simulink model "Example2"  (R2024b)
settings: Solver=FixedStepAuto  StartTime=0.0  StopTime=300  FixedStep=0.01  RelTol=1e-3
settings Model: Creator=aqx  LastModifiedBy=aqx
settings ModelReferenceCC: EnableRefExpFcnMdlSchedulingChecks=on
settings RTWCC: GPUComputeCapability=3.5

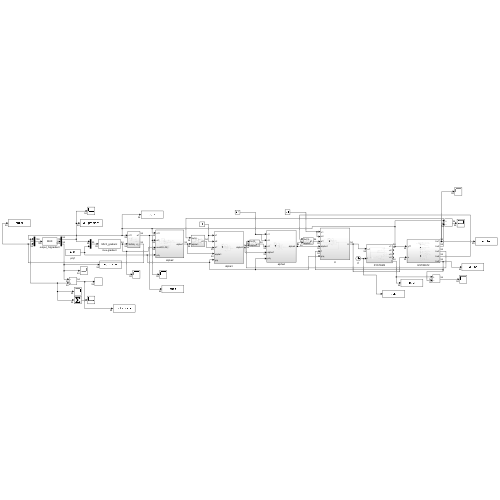
[thumbnail: Simulink's stored preview of the top-level diagram]
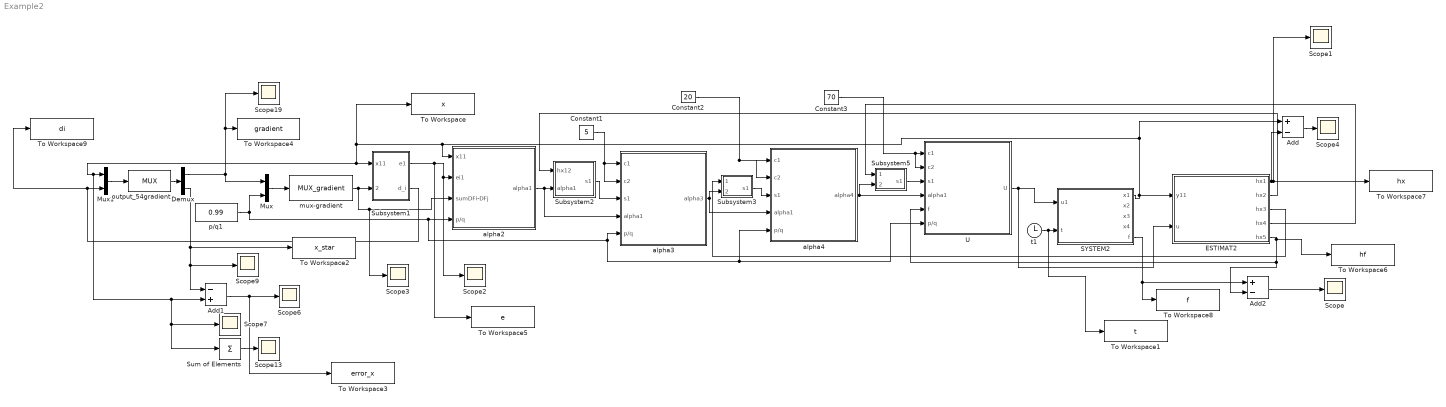
== system Example2 ==
  Add : Sum  Inputs=+-
  Add1 : Sum  Inputs=-+
  Add2 : Sum  Inputs=+-
  Constant1 : Constant  Value=5
  Constant2 : Constant  Value=20
  Constant3 : Constant  Value=70
  Demux : Demux  Outputs=2
  ESTIMAT2 : Subsystem
  Mux : Mux  Inputs=2
  Mux1 : Mux  Inputs=2
  SYSTEM2 : Subsystem
  Scope{,1..4,6..7,9,13,19} (10 alike) : Scope
  Subsystem1 : Subsystem
  Subsystem2 : Subsystem
  Subsystem3 : Subsystem
  Subsystem5 : Subsystem
  Sum of Elements : Sum  Inputs=+
  To Workspace : ToWorkspace  VariableName=x  SampleTime=-1
  To Workspace1 : ToWorkspace  VariableName=t  SampleTime=-1
  To Workspace2 : ToWorkspace  VariableName=x_star  SampleTime=-1
  To Workspace3 : ToWorkspace  VariableName=error_x  SampleTime=-1
  To Workspace4 : ToWorkspace  VariableName=gradient  SampleTime=-1
  To Workspace5 : ToWorkspace  VariableName=e  SampleTime=-1
  To Workspace6 : ToWorkspace  VariableName=hf  SampleTime=-1
  To Workspace7 : ToWorkspace  VariableName=hx  SampleTime=-1
  To Workspace8 : ToWorkspace  VariableName=f  SampleTime=-1
  To Workspace9 : ToWorkspace  VariableName=di  SampleTime=-1
  U : Subsystem
  alpha2 : Subsystem
  alpha3 : Subsystem
  alpha4 : Subsystem
  mux-gradient : S-Function  FunctionName=MUX_gradient  SFunctionDeploymentMode=off  EnableBusSupport=off
  output_54gradient : S-Function  FunctionName=MUX  SFunctionDeploymentMode=off  EnableBusSupport=off
  p/q1 : Constant  Value=0.99
  t1 : Clock
  wires:
  Mux/1 -> mux-gradient/1
  p/q1/1 -> U/6(p/q), alpha4/5(p/q), alpha3/5(p/q), alpha2/4(p/q), Mux/2
  mux-gradient/1 -> Scope3/1, alpha2/3(sumDFi-DFj), Subsystem1/2(SUMi-j)
  Subsystem1/1(e1) -> Scope2/1, alpha2/2(ei1), To Workspace5/1
  alpha2/1(alpha1) -> alpha3/4(alpha1), Subsystem2/2(alpha1)
  Subsystem2/1(s1) -> alpha3/3(s1)
  Constant1/1 -> alpha3/2(c2), alpha3/1(c1)
  t1/1 -> To Workspace1/1, SYSTEM2/2(t)
  SYSTEM2/1(x1) -> ESTIMAT2/1(y11), Add/1, To Workspace/1, Sum of Elements/1, Scope7/1, Add1/2, Mux1/1, Subsystem1/1(x11), alpha2/1(x11)
  Add/1 -> Scope4/1
  alpha3/1(alpha3) -> alpha4/4(alpha1), Subsystem3/2(alpha1)
  Subsystem3/1(s1) -> alpha4/3(s1)
  Mux1/1 -> output_54gradient/1
  Subsystem1/2(d_i) -> To Workspace9/1, Mux1/2
  output_54gradient/1 -> Demux/1
  Demux/1 -> Mux/1, Scope19/1, To Workspace4/1
  Demux/2 -> Add1/1, Scope9/1, To Workspace2/1
  Add1/1 -> To Workspace3/1, Scope6/1
  alpha4/1(alpha4) -> U/4(alpha1), Subsystem5/2(alpha1)
  Subsystem5/1(s1) -> U/3(s1)
  U/1(U) -> SYSTEM2/1(u1), ESTIMAT2/2(u)
  Constant3/1 -> U/2(c2), U/1(c1)
  Constant2/1 -> alpha4/2(c2), alpha4/1(c1)
  Sum of Elements/1 -> Scope13/1
  ESTIMAT2/1(hx1) -> Add/2, To Workspace7/1, Scope1/1
  ESTIMAT2/2(hx2) -> Subsystem2/1(hx12)
  ESTIMAT2/3(hx3) -> Subsystem3/1(hx13)
  ESTIMAT2/4(hx4) -> Subsystem5/1(hx13)
  ESTIMAT2/5(hx5) -> To Workspace6/1, Add2/2, U/5(f)
  SYSTEM2/5(f) -> To Workspace8/1, Add2/1
  Add2/1 -> Scope/1

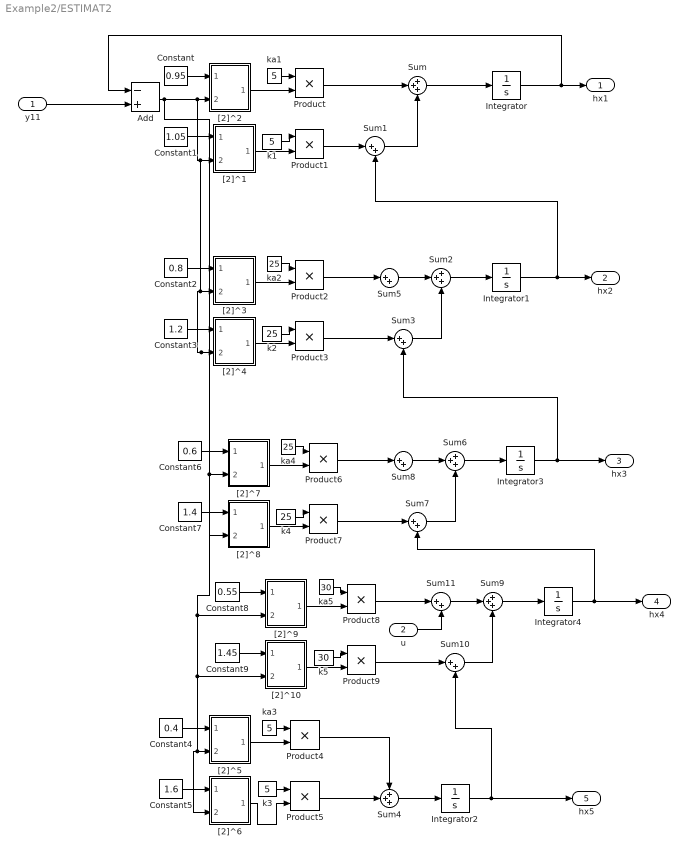
== system Example2/ESTIMAT2 ==
  y11 : Inport
  u : Inport  Port=2
  Add : Sum  Inputs=-+
  Constant : Constant  Value=0.95
  Constant1 : Constant  Value=1.05
  Constant2 : Constant  Value=0.8
  Constant3 : Constant  Value=1.2
  Constant4 : Constant  Value=0.4
  Constant5 : Constant  Value=1.6
  Constant6 : Constant  Value=0.6
  Constant7 : Constant  Value=1.4
  Constant8 : Constant  Value=0.55
  Constant9 : Constant  Value=1.45
  Integrator : Integrator  InitialCondition=45
  Integrator{1..4} (4 alike) : Integrator
  Product{,1..9} (10 alike) : Product
  Sum{,2,4,6,9} (5 alike) : Sum  Inputs=3
  Sum{1,3,5,7..8,10..11} (7 alike) : Sum  Inputs=|++
  "[2]^1" : Subsystem
  "[2]^10" : Subsystem
  "[2]^2" : Subsystem
  "[2]^3" : Subsystem
  "[2]^4" : Subsystem
  "[2]^5" : Subsystem
  "[2]^6" : Subsystem
  "[2]^7" : Subsystem
  "[2]^8" : Subsystem
  "[2]^9" : Subsystem
  k1 : Constant  Value=5
  k2 : Constant  Value=25
  k3 : Constant  Value=5
  k4 : Constant  Value=25
  k5 : Constant  Value=30
  ka1 : Constant  Value=5
  ka2 : Constant  Value=25
  ka3 : Constant  Value=5
  ka4 : Constant  Value=25
  ka5 : Constant  Value=30
  hx1 : Outport
  hx2 : Outport  Port=2
  hx3 : Outport  Port=3
  hx4 : Outport  Port=4
  hx5 : Outport  Port=5
  wires:
  Integrator/1 -> Add/1, hx1/1
  Sum1/1 -> Sum/3
  Sum/1 -> Integrator/1
  Integrator1/1 -> Sum1/2, hx2/1
  y11/1 -> Add/2
  "[2]^2"/1(Out1) -> Product/2
  "[2]^1"/1(Out1) -> Product1/2
  ka1/1 -> Product/1
  k1/1 -> Product1/1
  Product/1 -> Sum/2
  Product1/1 -> Sum1/1
  Sum2/1 -> Integrator1/1
  Sum3/1 -> Sum2/3
  Integrator2/1 -> hx5/1, Sum10/2
  ka2/1 -> Product2/1
  k2/1 -> Product3/1
  "[2]^4"/1(Out1) -> Product3/2
  "[2]^3"/1(Out1) -> Product2/2
  Product3/1 -> Sum3/1
  Sum4/1 -> Integrator2/1
  k3/1 -> Product5/1
  "[2]^6"/1(Out1) -> Product5/2
  ka3/1 -> Product4/1
  Add/1 -> "[2]^8"/2(In2), "[2]^7"/2(In2), "[2]^1"/2(In2), "[2]^3"/2(In2), "[2]^4"/2(In2), "[2]^9"/2(In2), "[2]^5"/2(In2), "[2]^6"/2(In2), "[2]^10"/2(In2), "[2]^2"/2(In2)
  "[2]^5"/1(Out1) -> Product4/2
  Product5/1 -> Sum4/2
  Product4/1 -> Sum4/1
  Product2/1 -> Sum5/1
  Sum5/1 -> Sum2/2
  Constant/1 -> "[2]^2"/1(In1)
  Constant1/1 -> "[2]^1"/1(In1)
  Constant2/1 -> "[2]^3"/1(In1)
  Constant3/1 -> "[2]^4"/1(In1)
  Constant4/1 -> "[2]^5"/1(In1)
  Constant5/1 -> "[2]^6"/1(In1)
  "[2]^8"/1(Out1) -> Product7/2
  Constant7/1 -> "[2]^8"/1(In1)
  Constant6/1 -> "[2]^7"/1(In1)
  "[2]^7"/1(Out1) -> Product6/2
  ka4/1 -> Product6/1
  Sum8/1 -> Sum6/2
  Sum6/1 -> Integrator3/1
  Product6/1 -> Sum8/1
  Integrator3/1 -> hx3/1, Sum3/2
  Product7/1 -> Sum7/1
  k4/1 -> Product7/1
  Sum7/1 -> Sum6/3
  k5/1 -> Product9/1
  Sum10/1 -> Sum9/3
  Product8/1 -> Sum11/1
  Product9/1 -> Sum10/1
  Integrator4/1 -> Sum7/2, hx4/1
  ka5/1 -> Product8/1
  Constant9/1 -> "[2]^10"/1(In1)
  Constant8/1 -> "[2]^9"/1(In1)
  Sum11/1 -> Sum9/2
  u/1 -> Sum11/2
  "[2]^9"/1(Out1) -> Product8/2
  Sum9/1 -> Integrator4/1
  "[2]^10"/1(Out1) -> Product9/2

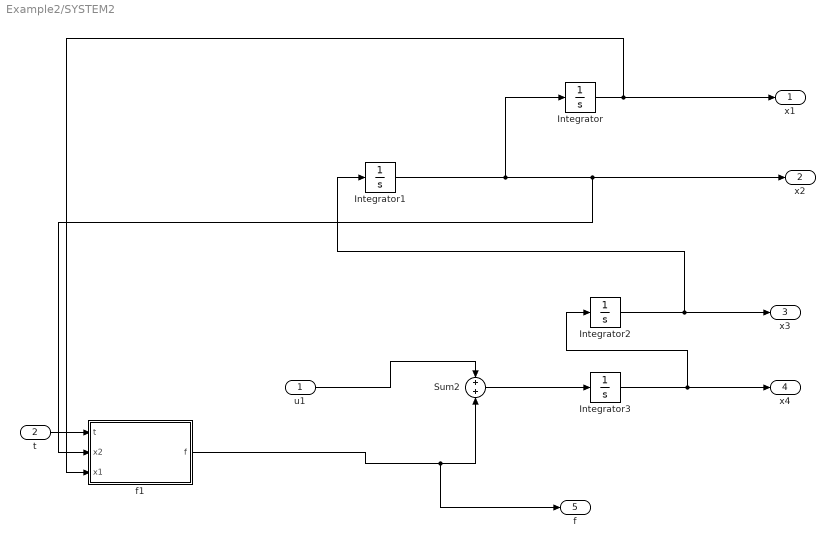
== system Example2/SYSTEM2 ==
  u1 : Inport
  t : Inport  Port=2
  Integrator : Integrator  InitialCondition=45
  Integrator1 : Integrator
  Integrator2 : Integrator
  Integrator3 : Integrator
  Sum2 : Sum  Inputs=2
  f1 : Subsystem
  x1 : Outport
  x2 : Outport  Port=2
  x3 : Outport  Port=3
  x4 : Outport  Port=4
  f : Outport  Port=5
  wires:
  Integrator/1 -> f1/3(x1), x1/1
  Integrator1/1 -> f1/2(x2), x2/1, Integrator/1
  Integrator2/1 -> Integrator1/1, x3/1
  f1/1(f) -> Sum2/2, f/1
  t/1 -> f1/1(t)
  Integrator3/1 -> Integrator2/1, x4/1
  Sum2/1 -> Integrator3/1
  u1/1 -> Sum2/1

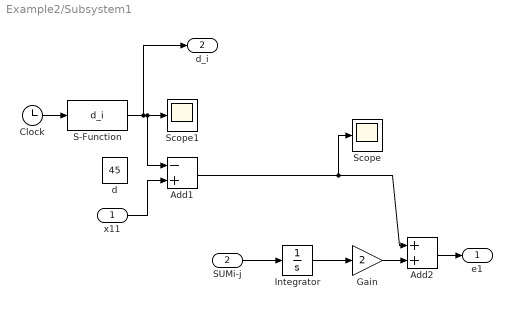
== system Example2/Subsystem1 ==
  x11 : Inport
  SUMi-j : Inport  Port=2
  Add1 : Sum  Inputs=-+
  Add2 : Sum
  Clock : Clock
  Gain : Gain  Gain=2
  Integrator : Integrator
  S-Function : S-Function  FunctionName=d_i  SFunctionDeploymentMode=off  EnableBusSupport=off
  Scope : Scope
  Scope1 : Scope
  d : Constant  Value=45
  e1 : Outport
  d_i : Outport  Port=2
  wires:
  x11/1 -> Add1/2
  SUMi-j/1 -> Integrator/1
  Integrator/1 -> Gain/1
  Gain/1 -> Add2/2
  Add1/1 -> Scope/1, Add2/1
  Add2/1 -> e1/1
  S-Function/1 -> d_i/1, Scope1/1, Add1/1
  Clock/1 -> S-Function/1

== system Example2/Subsystem2 ==
  hx12 : Inport
  alpha1 : Inport  Port=2
  Add : Sum  Inputs=+-
  Scope : Scope
  s1 : Outport
  wires:
  hx12/1 -> Add/1
  alpha1/1 -> Add/2
  Add/1 -> Scope/1, s1/1

== system Example2/Subsystem3 ==
  hx13 : Inport
  alpha1 : Inport  Port=2
  Add : Sum  Inputs=+-
  Scope : Scope
  s1 : Outport
  wires:
  hx13/1 -> Add/1
  alpha1/1 -> Add/2
  Add/1 -> Scope/1, s1/1

== system Example2/Subsystem5 ==
  hx13 : Inport
  alpha1 : Inport  Port=2
  Add : Sum  Inputs=+-
  Scope : Scope
  s1 : Outport
  wires:
  hx13/1 -> Add/1
  alpha1/1 -> Add/2
  Add/1 -> Scope/1, s1/1

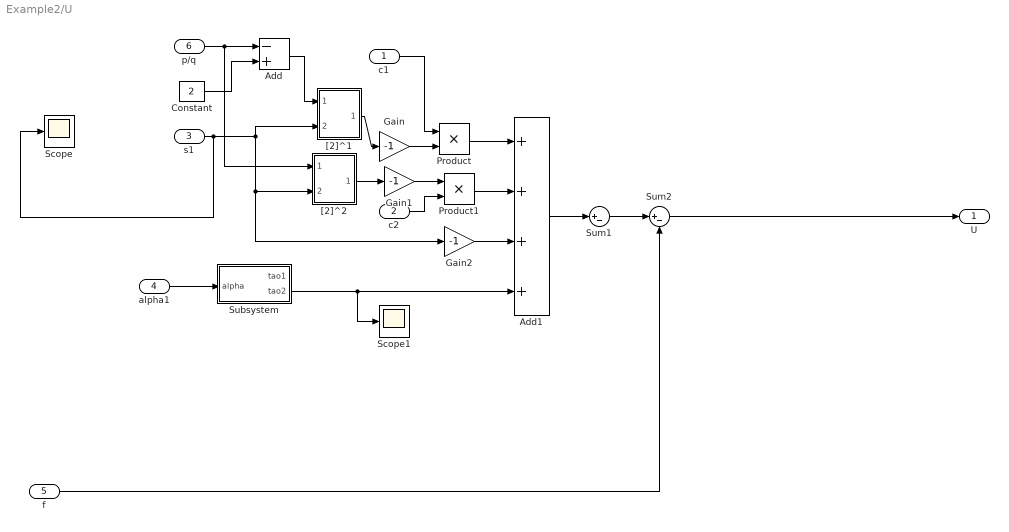
== system Example2/U ==
  c1 : Inport
  c2 : Inport  Port=2
  s1 : Inport  Port=3
  alpha1 : Inport  Port=4
  f : Inport  Port=5
  p/q : Inport  Port=6
  Add : Sum  Inputs=-+
  Add1 : Sum  Inputs=4
  Constant : Constant  Value=2
  Gain : Gain  Gain=-1
  Gain1 : Gain  Gain=-1
  Gain2 : Gain  Gain=-1
  Product : Product
  Product1 : Product
  Scope : Scope
  Scope1 : Scope
  Subsystem : Subsystem
  Sum1 : Sum  Inputs=|+-
  Sum2 : Sum  Inputs=|+-
  "[2]^1" : Subsystem
  "[2]^2" : Subsystem
  U : Outport
  wires:
  p/q/1 -> "[2]^2"/1(In1), Add/1
  Constant/1 -> Add/2
  s1/1 -> Scope/1, "[2]^2"/2(In2), Gain2/1, "[2]^1"/2(In2)
  Add/1 -> "[2]^1"/1(In1)
  "[2]^1"/1(Out1) -> Gain/1
  "[2]^2"/1(Out1) -> Gain1/1
  Gain/1 -> Product/2
  c1/1 -> Product/1
  Gain1/1 -> Product1/1
  c2/1 -> Product1/2
  alpha1/1 -> Subsystem/1(alpha)
  Product/1 -> Add1/1
  Product1/1 -> Add1/2
  Gain2/1 -> Add1/3
  Add1/1 -> Sum1/1
  Subsystem/2(tao2) -> Scope1/1, Add1/4
  Sum1/1 -> Sum2/1
  Sum2/1 -> U/1
  f/1 -> Sum2/2

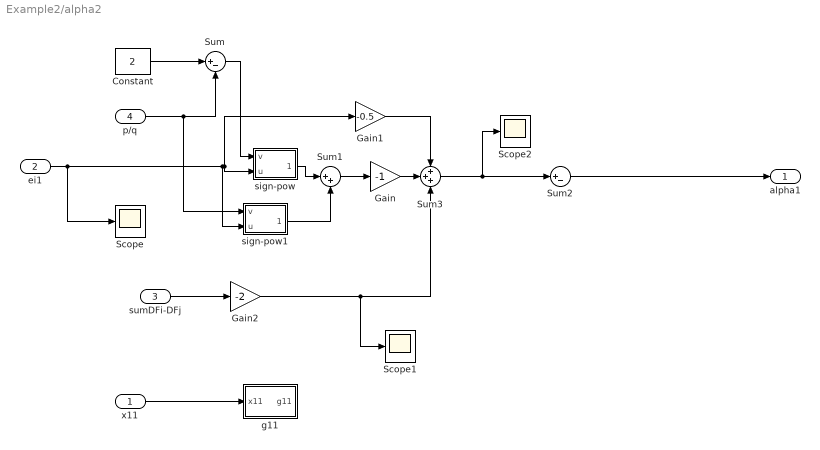
== system Example2/alpha2 ==
  x11 : Inport
  ei1 : Inport  Port=2
  sumDFi-DFj : Inport  Port=3
  p/q : Inport  Port=4
  Constant : Constant  Value=2
  Gain : Gain  Gain=-1
  Gain1 : Gain  Gain=-0.5
  Gain2 : Gain  Gain=-2
  Scope : Scope
  Scope1 : Scope
  Scope2 : Scope
  Sum : Sum  Inputs=|+-
  Sum1 : Sum  Inputs=|++
  Sum2 : Sum  Inputs=|+-
  Sum3 : Sum  Inputs=+++
  g11 : Subsystem
  sign-pow : Subsystem
  sign-pow1 : Subsystem
  alpha1 : Outport
  wires:
  Constant/1 -> Sum/1
  p/q/1 -> sign-pow1/1(v), Sum/2
  ei1/1 -> sign-pow1/2(u), Gain1/1, sign-pow/2(u), Scope/1
  Sum/1 -> sign-pow/1(v)
  sign-pow/1(Out1) -> Sum1/1
  sign-pow1/1(Out1) -> Sum1/2
  Sum1/1 -> Gain/1
  Gain/1 -> Sum3/2
  Sum3/1 -> Sum2/1, Scope2/1
  Gain1/1 -> Sum3/1
  sumDFi-DFj/1 -> Gain2/1
  x11/1 -> g11/1(x11)
  Sum2/1 -> alpha1/1
  Gain2/1 -> Scope1/1, Sum3/3

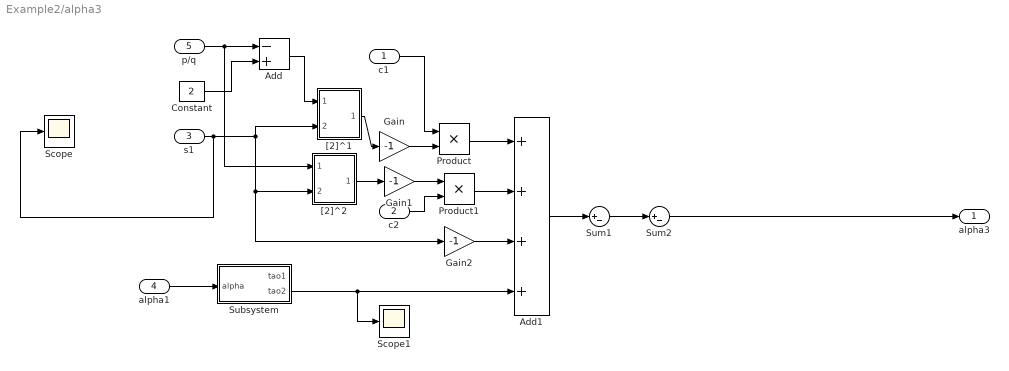
== system Example2/alpha3 ==
  c1 : Inport
  c2 : Inport  Port=2
  s1 : Inport  Port=3
  alpha1 : Inport  Port=4
  p/q : Inport  Port=5
  Add : Sum  Inputs=-+
  Add1 : Sum  Inputs=4
  Constant : Constant  Value=2
  Gain : Gain  Gain=-1
  Gain1 : Gain  Gain=-1
  Gain2 : Gain  Gain=-1
  Product : Product
  Product1 : Product
  Scope : Scope
  Scope1 : Scope
  Subsystem : Subsystem
  Sum1 : Sum  Inputs=|+-
  Sum2 : Sum  Inputs=|+-
  "[2]^1" : Subsystem
  "[2]^2" : Subsystem
  alpha3 : Outport
  wires:
  p/q/1 -> "[2]^2"/1(In1), Add/1
  Constant/1 -> Add/2
  s1/1 -> Scope/1, "[2]^2"/2(In2), Gain2/1, "[2]^1"/2(In2)
  Add/1 -> "[2]^1"/1(In1)
  "[2]^1"/1(Out1) -> Gain/1
  "[2]^2"/1(Out1) -> Gain1/1
  Gain/1 -> Product/2
  c1/1 -> Product/1
  Gain1/1 -> Product1/1
  c2/1 -> Product1/2
  alpha1/1 -> Subsystem/1(alpha)
  Product/1 -> Add1/1
  Product1/1 -> Add1/2
  Gain2/1 -> Add1/3
  Add1/1 -> Sum1/1
  Subsystem/2(tao2) -> Scope1/1, Add1/4
  Sum1/1 -> Sum2/1
  Sum2/1 -> alpha3/1

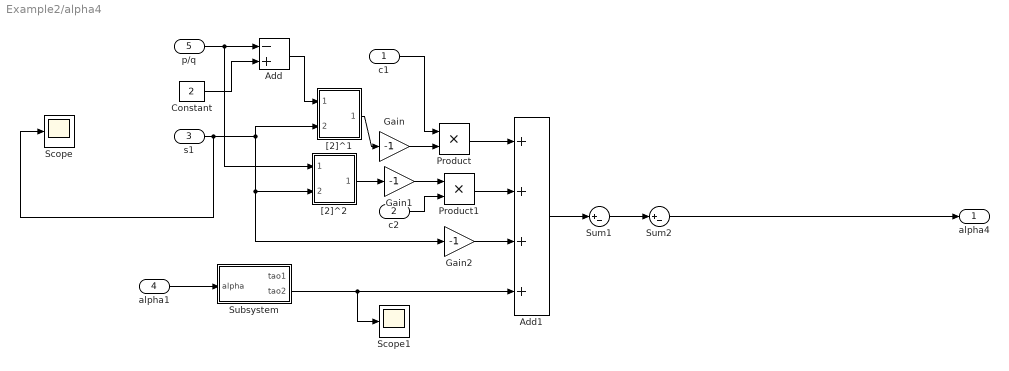
== system Example2/alpha4 ==
  c1 : Inport
  c2 : Inport  Port=2
  s1 : Inport  Port=3
  alpha1 : Inport  Port=4
  p/q : Inport  Port=5
  Add : Sum  Inputs=-+
  Add1 : Sum  Inputs=4
  Constant : Constant  Value=2
  Gain : Gain  Gain=-1
  Gain1 : Gain  Gain=-1
  Gain2 : Gain  Gain=-1
  Product : Product
  Product1 : Product
  Scope : Scope
  Scope1 : Scope
  Subsystem : Subsystem
  Sum1 : Sum  Inputs=|+-
  Sum2 : Sum  Inputs=|+-
  "[2]^1" : Subsystem
  "[2]^2" : Subsystem
  alpha4 : Outport
  wires:
  p/q/1 -> "[2]^2"/1(In1), Add/1
  Constant/1 -> Add/2
  s1/1 -> Scope/1, "[2]^2"/2(In2), Gain2/1, "[2]^1"/2(In2)
  Add/1 -> "[2]^1"/1(In1)
  "[2]^1"/1(Out1) -> Gain/1
  "[2]^2"/1(Out1) -> Gain1/1
  Gain/1 -> Product/2
  c1/1 -> Product/1
  Gain1/1 -> Product1/1
  c2/1 -> Product1/2
  alpha1/1 -> Subsystem/1(alpha)
  Product/1 -> Add1/1
  Product1/1 -> Add1/2
  Gain2/1 -> Add1/3
  Add1/1 -> Sum1/1
  Subsystem/2(tao2) -> Scope1/1, Add1/4
  Sum1/1 -> Sum2/1
  Sum2/1 -> alpha4/1

== system Example2/ESTIMAT2/[2]^1 ==
  In1 : Inport
  In2 : Inport  Port=2
  Pow : Math  Operator=pow  SignedPower=on  RndMeth=Zero
  Out1 : Outport
  wires:
  In2/1 -> Pow/1
  Pow/1 -> Out1/1
  In1/1 -> Pow/2

== system Example2/ESTIMAT2/[2]^10 ==
  In1 : Inport
  In2 : Inport  Port=2
  Pow : Math  Operator=pow  SignedPower=on  RndMeth=Zero
  Out1 : Outport
  wires:
  In2/1 -> Pow/1
  Pow/1 -> Out1/1
  In1/1 -> Pow/2

== system Example2/ESTIMAT2/[2]^2 ==
  In1 : Inport
  In2 : Inport  Port=2
  Pow : Math  Operator=pow  SignedPower=on  RndMeth=Zero
  Out1 : Outport
  wires:
  In2/1 -> Pow/1
  Pow/1 -> Out1/1
  In1/1 -> Pow/2

== system Example2/ESTIMAT2/[2]^3 ==
  In1 : Inport
  In2 : Inport  Port=2
  Pow : Math  Operator=pow  SignedPower=on  RndMeth=Zero
  Out1 : Outport
  wires:
  In2/1 -> Pow/1
  Pow/1 -> Out1/1
  In1/1 -> Pow/2

== system Example2/ESTIMAT2/[2]^4 ==
  In1 : Inport
  In2 : Inport  Port=2
  Pow : Math  Operator=pow  SignedPower=on  RndMeth=Zero
  Out1 : Outport
  wires:
  In2/1 -> Pow/1
  Pow/1 -> Out1/1
  In1/1 -> Pow/2

== system Example2/ESTIMAT2/[2]^5 ==
  In1 : Inport
  In2 : Inport  Port=2
  Pow : Math  Operator=pow  SignedPower=on  RndMeth=Zero
  Out1 : Outport
  wires:
  In2/1 -> Pow/1
  Pow/1 -> Out1/1
  In1/1 -> Pow/2

== system Example2/ESTIMAT2/[2]^6 ==
  In1 : Inport
  In2 : Inport  Port=2
  Pow : Math  Operator=pow  SignedPower=on  RndMeth=Zero
  Out1 : Outport
  wires:
  In2/1 -> Pow/1
  Pow/1 -> Out1/1
  In1/1 -> Pow/2

== system Example2/ESTIMAT2/[2]^7 ==
  In1 : Inport
  In2 : Inport  Port=2
  Pow : Math  Operator=pow  SignedPower=on  RndMeth=Zero
  Out1 : Outport
  wires:
  In2/1 -> Pow/1
  Pow/1 -> Out1/1
  In1/1 -> Pow/2

== system Example2/ESTIMAT2/[2]^8 ==
  In1 : Inport
  In2 : Inport  Port=2
  Pow : Math  Operator=pow  SignedPower=on  RndMeth=Zero
  Out1 : Outport
  wires:
  In2/1 -> Pow/1
  Pow/1 -> Out1/1
  In1/1 -> Pow/2

== system Example2/ESTIMAT2/[2]^9 ==
  In1 : Inport
  In2 : Inport  Port=2
  Pow : Math  Operator=pow  SignedPower=on  RndMeth=Zero
  Out1 : Outport
  wires:
  In2/1 -> Pow/1
  Pow/1 -> Out1/1
  In1/1 -> Pow/2

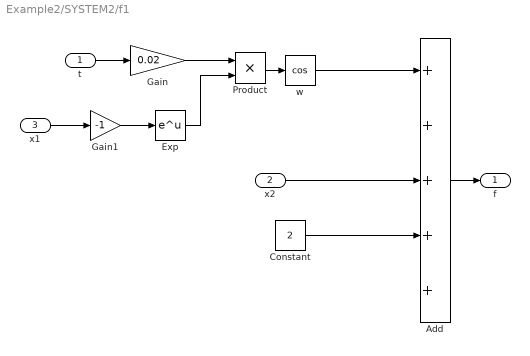
== system Example2/SYSTEM2/f1 ==
  t : Inport
  x2 : Inport  Port=2
  x1 : Inport  Port=3
  Add : Sum  Inputs=5
  Constant : Constant  Value=2
  Exp : Math
  Gain : Gain  Gain=0.02
  Gain1 : Gain  Gain=-1
  Product : Product
  w : Trigonometry  Operator=cos
  f : Outport
  wires:
  Add/1 -> f/1
  x1/1 -> Gain1/1
  Constant/1 -> Add/4
  t/1 -> Gain/1
  w/1 -> Add/1
  Product/1 -> w/1
  Gain/1 -> Product/1
  Exp/1 -> Product/2
  Gain1/1 -> Exp/1
  x2/1 -> Add/3

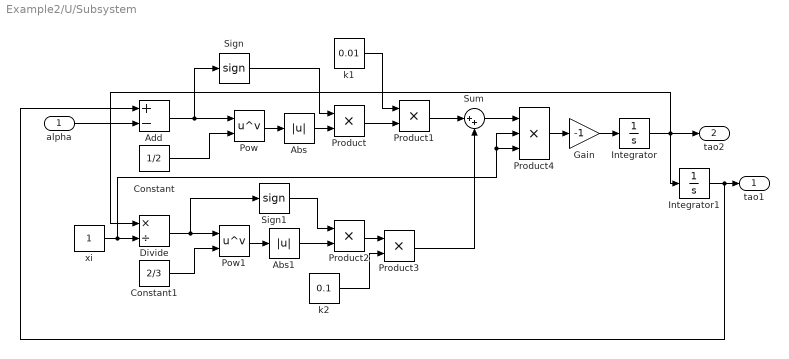
== system Example2/U/Subsystem ==
  alpha : Inport
  Abs : Abs  SaturateOnIntegerOverflow=off
  Abs1 : Abs  SaturateOnIntegerOverflow=off
  Add : Sum  Inputs=+-
  Constant : Constant  Value=1/2
  Constant1 : Constant  Value=2/3
  Divide : Product  Inputs=*/
  Gain : Gain  Gain=-1
  Integrator : Integrator
  Integrator1 : Integrator
  Pow : Math  Operator=pow  SignedPower=on  RndMeth=Zero
  Pow1 : Math  Operator=pow  SignedPower=on  RndMeth=Zero
  Product{,1..3} (4 alike) : Product
  Product4 : Product  Inputs=3
  Sign : Signum
  Sign1 : Signum
  Sum : Sum  Inputs=|++
  k1 : Constant  Value=0.01
  k2 : Constant  Value=0.1
  xi : Constant
  tao1 : Outport
  tao2 : Outport  Port=2
  wires:
  alpha/1 -> Add/2
  Add/1 -> Pow/1, Sign/1
  Constant/1 -> Pow/2
  Pow/1 -> Abs/1
  Abs/1 -> Product/2
  Sign/1 -> Product/1
  Product/1 -> Product1/2
  k1/1 -> Product1/1
  Product1/1 -> Sum/1
  xi/1 -> Product4/2, Product4/3, Divide/2
  Divide/1 -> Sign1/1, Pow1/1
  Constant1/1 -> Pow1/2
  Pow1/1 -> Abs1/1
  Abs1/1 -> Product2/2
  Sign1/1 -> Product2/1
  Product2/1 -> Product3/1
  k2/1 -> Product3/2
  Product3/1 -> Sum/2
  Sum/1 -> Product4/1
  Product4/1 -> Gain/1
  Gain/1 -> Integrator/1
  Integrator/1 -> Divide/1, Integrator1/1, tao2/1
  Integrator1/1 -> Add/1, tao1/1

== system Example2/U/[2]^1 ==
  In1 : Inport
  In2 : Inport  Port=2
  Pow : Math  Operator=pow  SignedPower=on  RndMeth=Zero
  Out1 : Outport
  wires:
  In2/1 -> Pow/1
  Pow/1 -> Out1/1
  In1/1 -> Pow/2

== system Example2/U/[2]^2 ==
  In1 : Inport
  In2 : Inport  Port=2
  Pow : Math  Operator=pow  SignedPower=on  RndMeth=Zero
  Out1 : Outport
  wires:
  In2/1 -> Pow/1
  Pow/1 -> Out1/1
  In1/1 -> Pow/2

== system Example2/alpha2/g11 ==
  x11 : Inport
  Cos : Trigonometry  Operator=cos
  Sum : Sum  Inputs=|++
  g11 : Outport
  wires:
  Cos/1 -> Sum/1
  Sum/1 -> g11/1
  x11/1 -> Sum/2, Cos/1

== system Example2/alpha2/sign-pow ==
  v : Inport
  u : Inport  Port=2
  Abs : Abs  SaturateOnIntegerOverflow=off
  Pow : Math  Operator=pow  SignedPower=on  RndMeth=Zero
  Product : Product
  signn : Subsystem
  Out1 : Outport
  wires:
  u/1 -> signn/1(In1), Abs/1
  Abs/1 -> Pow/1
  v/1 -> Pow/2
  Pow/1 -> Product/2
  signn/1(Out1) -> Product/1
  Product/1 -> Out1/1

== system Example2/alpha2/sign-pow1 ==
  v : Inport
  u : Inport  Port=2
  Abs : Abs  SaturateOnIntegerOverflow=off
  Pow : Math  Operator=pow  SignedPower=on  RndMeth=Zero
  Product : Product
  signn : Subsystem
  Out1 : Outport
  wires:
  u/1 -> signn/1(In1), Abs/1
  Abs/1 -> Pow/1
  v/1 -> Pow/2
  Pow/1 -> Product/2
  signn/1(Out1) -> Product/1
  Product/1 -> Out1/1

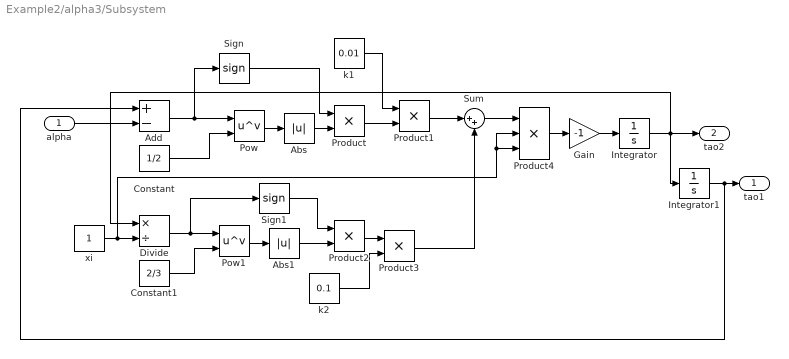
== system Example2/alpha3/Subsystem ==
  alpha : Inport
  Abs : Abs  SaturateOnIntegerOverflow=off
  Abs1 : Abs  SaturateOnIntegerOverflow=off
  Add : Sum  Inputs=+-
  Constant : Constant  Value=1/2
  Constant1 : Constant  Value=2/3
  Divide : Product  Inputs=*/
  Gain : Gain  Gain=-1
  Integrator : Integrator
  Integrator1 : Integrator
  Pow : Math  Operator=pow  SignedPower=on  RndMeth=Zero
  Pow1 : Math  Operator=pow  SignedPower=on  RndMeth=Zero
  Product{,1..3} (4 alike) : Product
  Product4 : Product  Inputs=3
  Sign : Signum
  Sign1 : Signum
  Sum : Sum  Inputs=|++
  k1 : Constant  Value=0.01
  k2 : Constant  Value=0.1
  xi : Constant
  tao1 : Outport
  tao2 : Outport  Port=2
  wires:
  alpha/1 -> Add/2
  Add/1 -> Pow/1, Sign/1
  Constant/1 -> Pow/2
  Pow/1 -> Abs/1
  Abs/1 -> Product/2
  Sign/1 -> Product/1
  Product/1 -> Product1/2
  k1/1 -> Product1/1
  Product1/1 -> Sum/1
  xi/1 -> Product4/2, Product4/3, Divide/2
  Divide/1 -> Sign1/1, Pow1/1
  Constant1/1 -> Pow1/2
  Pow1/1 -> Abs1/1
  Abs1/1 -> Product2/2
  Sign1/1 -> Product2/1
  Product2/1 -> Product3/1
  k2/1 -> Product3/2
  Product3/1 -> Sum/2
  Sum/1 -> Product4/1
  Product4/1 -> Gain/1
  Gain/1 -> Integrator/1
  Integrator/1 -> Divide/1, Integrator1/1, tao2/1
  Integrator1/1 -> Add/1, tao1/1

== system Example2/alpha3/[2]^1 ==
  In1 : Inport
  In2 : Inport  Port=2
  Pow : Math  Operator=pow  SignedPower=on  RndMeth=Zero
  Out1 : Outport
  wires:
  In2/1 -> Pow/1
  Pow/1 -> Out1/1
  In1/1 -> Pow/2

== system Example2/alpha3/[2]^2 ==
  In1 : Inport
  In2 : Inport  Port=2
  Pow : Math  Operator=pow  SignedPower=on  RndMeth=Zero
  Out1 : Outport
  wires:
  In2/1 -> Pow/1
  Pow/1 -> Out1/1
  In1/1 -> Pow/2

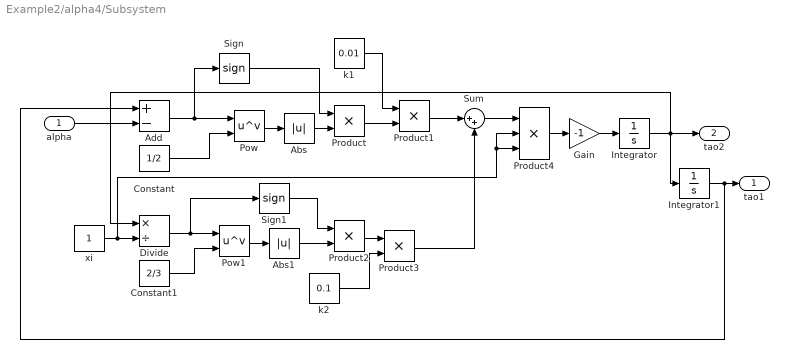
== system Example2/alpha4/Subsystem ==
  alpha : Inport
  Abs : Abs  SaturateOnIntegerOverflow=off
  Abs1 : Abs  SaturateOnIntegerOverflow=off
  Add : Sum  Inputs=+-
  Constant : Constant  Value=1/2
  Constant1 : Constant  Value=2/3
  Divide : Product  Inputs=*/
  Gain : Gain  Gain=-1
  Integrator : Integrator
  Integrator1 : Integrator
  Pow : Math  Operator=pow  SignedPower=on  RndMeth=Zero
  Pow1 : Math  Operator=pow  SignedPower=on  RndMeth=Zero
  Product{,1..3} (4 alike) : Product
  Product4 : Product  Inputs=3
  Sign : Signum
  Sign1 : Signum
  Sum : Sum  Inputs=|++
  k1 : Constant  Value=0.01
  k2 : Constant  Value=0.1
  xi : Constant
  tao1 : Outport
  tao2 : Outport  Port=2
  wires:
  alpha/1 -> Add/2
  Add/1 -> Pow/1, Sign/1
  Constant/1 -> Pow/2
  Pow/1 -> Abs/1
  Abs/1 -> Product/2
  Sign/1 -> Product/1
  Product/1 -> Product1/2
  k1/1 -> Product1/1
  Product1/1 -> Sum/1
  xi/1 -> Product4/2, Product4/3, Divide/2
  Divide/1 -> Sign1/1, Pow1/1
  Constant1/1 -> Pow1/2
  Pow1/1 -> Abs1/1
  Abs1/1 -> Product2/2
  Sign1/1 -> Product2/1
  Product2/1 -> Product3/1
  k2/1 -> Product3/2
  Product3/1 -> Sum/2
  Sum/1 -> Product4/1
  Product4/1 -> Gain/1
  Gain/1 -> Integrator/1
  Integrator/1 -> Divide/1, Integrator1/1, tao2/1
  Integrator1/1 -> Add/1, tao1/1

== system Example2/alpha4/[2]^1 ==
  In1 : Inport
  In2 : Inport  Port=2
  Pow : Math  Operator=pow  SignedPower=on  RndMeth=Zero
  Out1 : Outport
  wires:
  In2/1 -> Pow/1
  Pow/1 -> Out1/1
  In1/1 -> Pow/2

== system Example2/alpha4/[2]^2 ==
  In1 : Inport
  In2 : Inport  Port=2
  Pow : Math  Operator=pow  SignedPower=on  RndMeth=Zero
  Out1 : Outport
  wires:
  In2/1 -> Pow/1
  Pow/1 -> Out1/1
  In1/1 -> Pow/2

== system Example2/alpha2/sign-pow/signn ==
  In1 : Inport
  Constant3 : Constant  Value=4
  Constant4 : Constant
  Divide : Product  Inputs=*/
  Exp : Math
  Product : Product
  Sum5 : Sum  Inputs=|-+
  Sum6 : Sum  Inputs=|++
  Out1 : Outport
  wires:
  In1/1 -> Product/1
  Sum5/1 -> Divide/1
  Sum6/1 -> Divide/2
  Product/1 -> Exp/1
  Constant3/1 -> Product/2
  Exp/1 -> Sum6/1, Sum5/2
  Constant4/1 -> Sum5/1, Sum6/2
  Divide/1 -> Out1/1

== system Example2/alpha2/sign-pow1/signn ==
  In1 : Inport
  Constant3 : Constant  Value=4
  Constant4 : Constant
  Divide : Product  Inputs=*/
  Exp : Math
  Product : Product
  Sum5 : Sum  Inputs=|-+
  Sum6 : Sum  Inputs=|++
  Out1 : Outport
  wires:
  In1/1 -> Product/1
  Sum5/1 -> Divide/1
  Sum6/1 -> Divide/2
  Product/1 -> Exp/1
  Constant3/1 -> Product/2
  Exp/1 -> Sum6/1, Sum5/2
  Constant4/1 -> Sum5/1, Sum6/2
  Divide/1 -> Out1/1
